simulink model "MPPT_Efficiency_votlage_controlled"  (R2024b)
settings: Solver=FixedStepAuto  StartTime=0.0  StopTime=92  FixedStep=1e-6  RelTol=1e-3
libraries: spsSeriesRLCBranchLib x2, spsControlledVoltageSourceLib x1, spsCurrentMeasurementLib x1, spsGroundLib x1, spsPVArrayLib x1, SignalEditorBlockLib x1, spsVoltageMeasurementLib x1, sps_lib x1
settings Model: Creator=ethan  LastModifiedBy=ethan

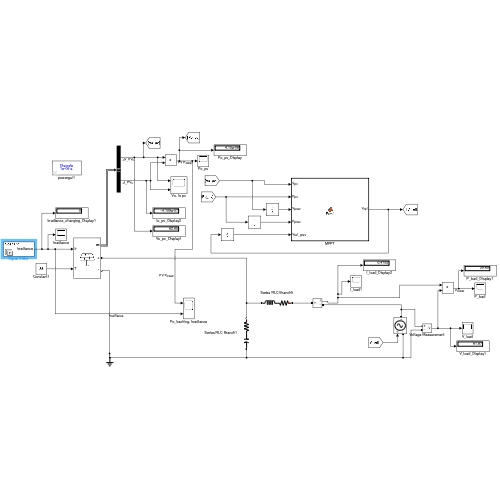
[thumbnail: Simulink's stored preview of the top-level diagram]
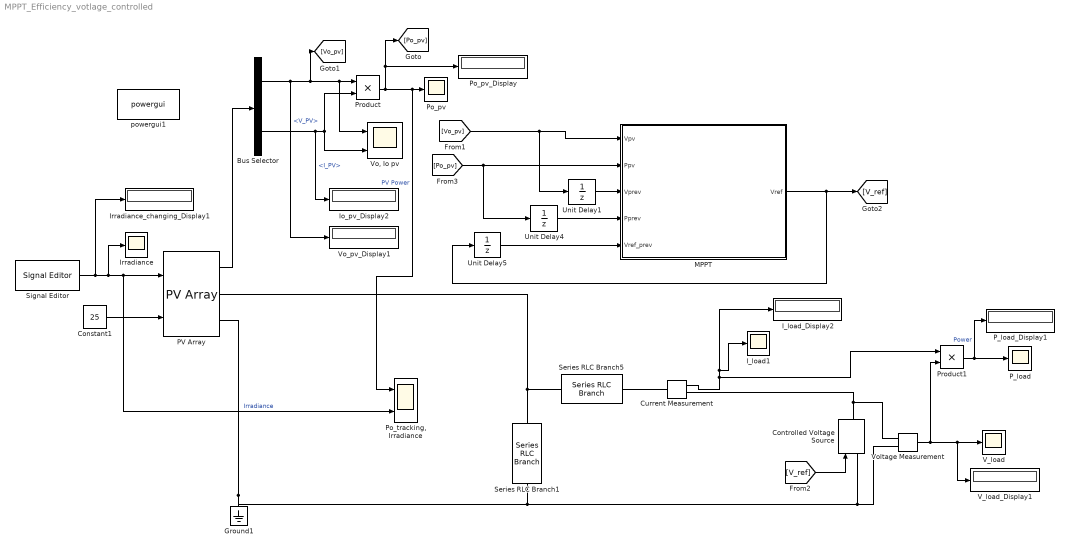
== system MPPT_Efficiency_votlage_controlled ==
  Bus Selector : BusSelector  OutputSignals=V_PV,I_PV
  Constant1 : Constant  Value=25
  Controlled Voltage Source : spsControlledVoltageSourceLib/Controlled Voltage Source  Initialize=on  Source_Type=DC  Amplitude=0  Phase=0  Frequency=0  Measurements=None
  Current Measurement : spsCurrentMeasurementLib/Current Measurement  PhasorSimulation=off  OutputType=Complex  PSBequivalent=0
  Ground1 : spsGroundLib/Ground  LConnTagsString=a
  I_load1 : Scope
  I_load_Display2 : Display
  Io_pv_Display2 : Display
  Irradiance : Scope
  Irradiance_changing_Display1 : Display
  MPPT : MATLAB Function  TreatAsAtomicUnit=on
  PV Array : spsPVArrayLib/PV Array  Npar=2  Nser=16  PlotType=array @ 25 deg.C & specified irradiances  S_vec=[ 1000 500 ]  Temp_C_vec="[ 25  ]"  ModuleName=User-defined  PlotWhenSelected=off  Pm=200.032  Ncell=70  Voc=45.3  Isc=5.84  Vm=37.6  Im=5.32  beta_Voc_pc=-0.2810  alpha_Isc_pc=0.0373  beta_Voc=-0.12729  alpha_Isc=0.0021783  IL=5.8604  I0=8.4912e-12  nI=0.92602  Rsh=133.307  Rs=0.46546  RobustModel=off  RobustCellTemperature=313.3991  BAL=on  Tc=1e-6  Tfilter=5e-5
  P_load : Scope
  P_load_Display1 : Display
  Po_pv : Scope
  Po_pv_Display : Display
  "Po_tracking, Irradiance" : Scope  NumInputPorts=2
  Product : Product
  Product1 : Product
  Series RLC Branch1 : spsSeriesRLCBranchLib/Series RLC Branch  LConnTagsString=__new0  RConnTagsString=__new0  BranchType=RC  Resistance=0.5  Inductance=2e-3  SetiL0=off  InitialCurrent=0  Capacitance=100e-6  Setx0=off  InitialVoltage=0  Measurements=None
  Series RLC Branch5 : spsSeriesRLCBranchLib/Series RLC Branch  LConnTagsString=__new0  RConnTagsString=__new0  BranchType=RL  Resistance=0.001  Inductance=1e-3  SetiL0=off  InitialCurrent=0  Capacitance=220e-6  Setx0=off  InitialVoltage=0  Measurements=None
  Signal Editor : SignalEditorBlockLib/Signal Editor  FileName=/Users/ethan/MATLAB-Drive/Irradiance.mat  ActiveScenario=Scenario  ActiveSignal=Irradiance  IsBus=off  OutputBusObjectStr=Bus: BusObject  SampleTime=0  ZeroCross=off  OutputAfterFinalValue=Setting to zero  Unit=inherit  PreserveSignalName=on  ApplySigPropsToAllScenarios=on  ApplySigPropsToAllSignals=on
  Unit Delay1 : UnitDelay  SampleTime=-1  HasFrameUpgradeWarning=on
  Unit Delay4 : UnitDelay  SampleTime=-1  HasFrameUpgradeWarning=on
  Unit Delay5 : UnitDelay  SampleTime=-1  HasFrameUpgradeWarning=on
  V_load : Scope
  V_load_Display1 : Display
  "Vo, Io pv" : Scope  NumInputPorts=2
  Vo_pv_Display1 : Display
  Voltage Measurement : spsVoltageMeasurementLib/Voltage Measurement  PhasorSimulation=off  OutputType=Complex  PSBequivalent=0
  powergui1 : sps_lib/powergui  Priority=1  SimulationMode=Discrete  SampleTime=1e-6  frequency=60  Iterations=50  frequencyindice=0  Pbase=100e6  ErrMax=1e-4  UnitsV=kV  UnitsW=MW  buscounter=0  FunctionMessages=off  echomessages=off  EnableUseOfTLC=off  CurrentSourceSwitches=off  DisableSnubberDevices=off  DisableRonSwitches=off  DisableVfSwitches=off  DisplayEquations=off  AutomaticDiscreteSolvers=off  SolverType=Tustin  Interpol=on  ExternalGateDelay=off  methode=off  Ts=100  x0status=blocks  SPID=on  SwTol=0  HookPort=off  NonlinearTolerance=1e-4  nMaxIteration=100  ContinueOnMaxIteration=off  RestoreLinks=warning  ResistiveCurrentMeasurement=off  Frange=[0:2:500]  Ylog=off  Xlog=on  ShowGrid=off  save=off  variable=ZData  structure=0  ZoomFFT=off  StartTime=0.0  cycles=1  DisplayStyle=1  fundamental=60  FreqAxis=off  MaxFrequency=1000  frequencyindicesteady=1  RmsSteady=1  display=off
  wires:
  Constant1/1 -> PV Array/2
  PV Array/1 -> Bus Selector/1
  Bus Selector/2 -> Io_pv_Display2/1, "Vo, Io pv"/2, Product/2  "<I_PV>"
  Bus Selector/1 -> Vo_pv_Display1/1, [Vo_pv], "Vo, Io pv"/1, Product/1  "<V_PV>"
  Product/1 -> [Po_pv], Po_pv_Display/1, "Po_tracking, Irradiance"/1, Po_pv/1  "PV Power"
  Unit Delay1/1 -> MPPT/3(Vprev)
  [Po_pv] -> Unit Delay4/1, MPPT/2(Ppv)
  Unit Delay4/1 -> MPPT/4(Pprev)
  MPPT/1(Vref) -> [V_ref], Unit Delay5/1
  [Vo_pv] -> Unit Delay1/1, MPPT/1(Vpv)
  Unit Delay5/1 -> MPPT/5(Vref_prev)
  [V_ref] -> Controlled Voltage Source/1
  Current Measurement/1 -> Product1/1, I_load_Display2/1, I_load1/1
  Voltage Measurement/1 -> V_load_Display1/1, V_load/1, Product1/2
  Product1/1 -> P_load_Display1/1, P_load/1  "Power"
  Signal Editor/1 -> Irradiance/1, "Po_tracking, Irradiance"/2, PV Array/1, Irradiance_changing_Display1/1  "Irradiance"
  connections:
  PV Array/RConn1 -- Series RLC Branch5/RConn1 -- Series RLC Branch1/LConn1
  Ground1/LConn1 -- Series RLC Branch1/RConn1 -- Controlled Voltage Source/LConn1 -- Voltage Measurement/LConn2 -- PV Array/RConn2
  Series RLC Branch5/LConn1 -- Current Measurement/LConn1
  Current Measurement/RConn1 -- Voltage Measurement/LConn1 -- Controlled Voltage Source/RConn1

== matlab function MPPT_Efficiency_votlage_controlled/MPPT ==
  data: Vpv input; Vref output; Ppv input; Vprev input; Pprev input; Vref_prev input
function Vref = fVref(Vpv, Ppv, Vprev, Pprev, Vref_prev)

% --- Parameters --------------------------------------------------
dV_step = 0.002;          % Voltage perturbation magnitude [V]
Vmin    = 0;            % Minimum allowed voltage reference [V]
Vmax    = 800;           % Maximum allowed voltage reference [V] 

% --- Initialisation (first call) ---------------------------------
if isempty(Vref_prev)
    Vref_prev = 600;   
end

% --- P&O Decision Logic ------------------------------------------
dP = Ppv - Pprev;       % change in power
dV = Vpv - Vprev;       % change in voltage

if dP > 0
    % Power increased → keep moving in same direction
    if dV > 0
        Vref = Vref_prev + dV_step;   % +dV gave +dP → continue increasing
    else
        Vref = Vref_prev - dV_step;   % -dV gave +dP → continue decreasing
    end
else
    % Power decreased → reverse direction
    if dV > 0
        Vref = Vref_prev - dV_step;   % +dV gave -dP → reverse, so decrease
    else
        Vref = Vref_prev + dV_step;   % -dV gave -dP → reverse, so increase
    end
end

% --- Enforce bounds ----------------------------------------------
Vref = max(min(Vref, Vmax), Vmin);

end
